simulink model "pendule_inv_etu"  (R2022b)
settings: Solver=VariableStepAuto  StartTime=0.0  StopTime=10.0  RelTol=1e-3
undefined symbols (not defined in the file): g, K, l, ue, x0, xe
settings Model: Creator=mathissigier  LastModifiedBy=mathissigier

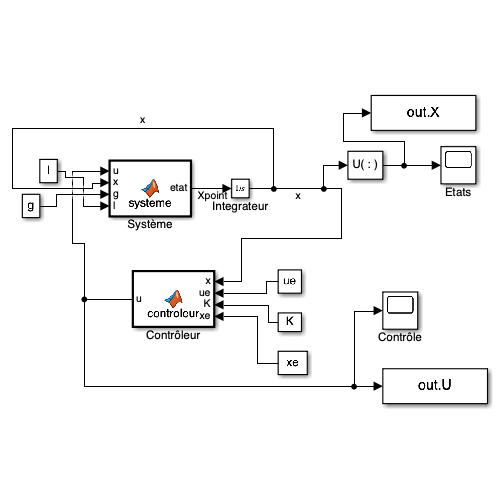
[thumbnail: Simulink's stored preview of the top-level diagram]
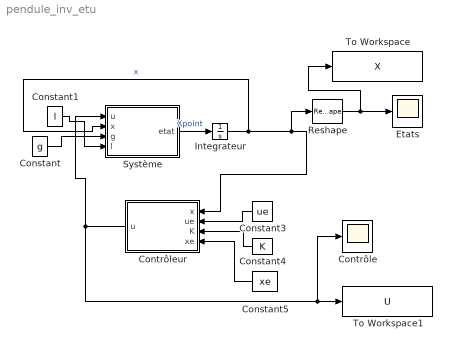
== system pendule_inv_etu ==
  Constant : Constant  Value=g
  Constant1 : Constant  Value=l
  Constant3 : Constant  Value=ue
  Constant4 : Constant  Value=K  VectorParams1D=off
  Constant5 : Constant  Value=xe  VectorParams1D=off
  Contrôle : Scope
  Contrôleur : MATLAB Function  TreatAsAtomicUnit=on
  Etats : Scope
      settings: Description=Etats
  Integrateur : Integrator  InitialCondition=x0
  Reshape : Reshape
  Système : MATLAB Function  TreatAsAtomicUnit=on
  To Workspace : ToWorkspace  VariableName=X  SaveFormat=Timeseries  SampleTime=-1
  To Workspace1 : ToWorkspace  VariableName=U  SaveFormat=Timeseries  SampleTime=-1
  wires:
  Contrôleur/1(u) -> Système/1(u), To Workspace1/1, Contrôle/1
  Constant/1 -> Système/3(g)
  Constant1/1 -> Système/4(l)
  Constant3/1 -> Contrôleur/2(ue)
  Constant4/1 -> Contrôleur/3(K)
  Constant5/1 -> Contrôleur/4(xe)
  Système/1(etat) -> Integrateur/1  "Xpoint"
  Integrateur/1 -> Système/2(x), Reshape/1, Contrôleur/1(x)  "x"
  Reshape/1 -> To Workspace/1, Etats/1

== matlab function pendule_inv_etu/Contrôleur ==
  data: x input; u output; ue input; K input; xe input
function u = controleur(x,ue,K,xe)

u = ue + K(:)'*(x-xe);

== matlab function pendule_inv_etu/Système ==
  data: u input; x input; etat output; g input; l input
function etat = systeme(u,x,g,l)

etat=[x(2);(g/l)*sin(x(1))-(u/l)*cos(x(1))];
